simulink model "hdlcoder_led_blinking_4bit"  (R2021b)
settings: Solver=FixedStepDiscrete  StartTime=0.0  StopTime=1  RelTol=1e-3
InitFcn:
  | Ts = 1e-3;
libraries: hdlsllib x3, simulink x2
settings Model: Creator=The MathWorks, Inc.  LastModifiedBy=Jeedella
settings SolverCC: AlgebraicLoopSolver=TrustRegion
settings DataIOCC: LimitDataPoints=on  SaveFormat=Array  SaveOutput=off  SignalLogging=off  SaveTime=off  ReturnWorkspaceOutputs=off
settings OptimizationCC: BlockReduction=off  ConditionallyExecuteInputs=off  DefaultParameterBehavior=Inlined  ExpressionDepthLimit=2147483647  LifeSpan=inf
settings DebuggingCC: AlgebraicLoopMsg=error  UnderspecifiedInitializationDetection=Classic  MergeDetectMultiDrivingBlocksExec=none  SolverPrmCheckMsg=warning  SingleTaskRateTransMsg=error  ParameterPrecisionLossMsg=none  StateNameClashWarn=warning  SFUnexpectedBacktrackingDiag=warning  SFNoUnconditionalDefaultTransitionDiag=warning  SFExecutionAtInitializationDiag=none  SFMachineParentedDataDiag=warning  ArithmeticOperatorsInVariantConditions=warning
settings HardwareCC: ProdBitPerPointer=32  ProdBitPerSizeT=32  ProdBitPerPtrDiffT=32  ProdLargestAtomicFloat=None  ProdIntDivRoundTo=Undefined  ProdEndianess=Unspecified  ProdWordSize=32  ProdHWDeviceType=ASIC/FPGA->ASIC/FPGA  ProdEqTarget=off
settings ModelReferenceCC: PropagateSignalLabelsOutOfModel=off
settings SFSimCC: SimUseLocalCustomCode=off  CustomCodeUndefinedFunction=UseInterfaceOnly
settings RTWCC: RTWUseLocalCustomCode=off
settings CodeAppCC: StateflowObjectComments=on
settings GRTTargetCC: TargetLangStandard=C89/C90 (ANSI)
settings ConfigComp: CovMetricSettings=dw  CovSaveCumulativeToWorkspaceVar=on  CovSaveSingleToWorkspaceVar=on  CovExternalEMLEnable=off  CovSFcnEnable=off

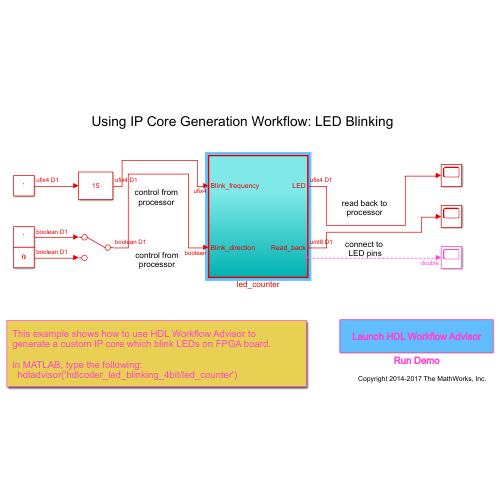
[thumbnail: Simulink's stored preview of the top-level diagram]
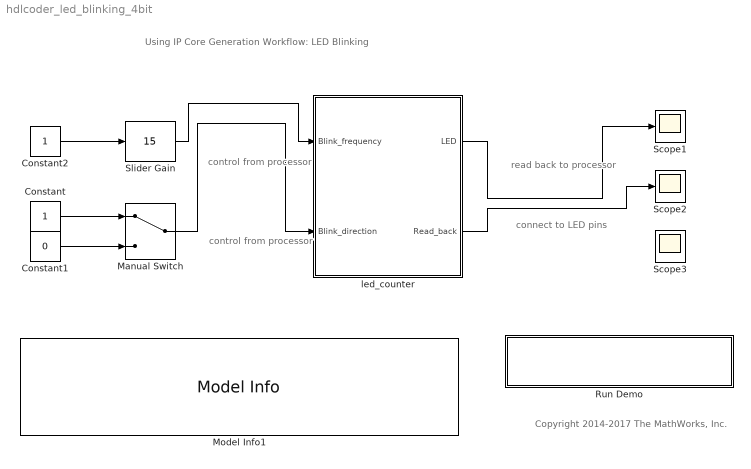
== system hdlcoder_led_blinking_4bit ==
  note: control from
      | processor
  note: Copyright 2014-2017 The MathWorks, Inc.
  note: Using IP Core Generation Workflow: LED Blinking
  note: control from
      | processor
  note: read back to
      | processor
  note: connect to
      | LED pins
  Constant : Constant  OutDataTypeStr=boolean  SampleTime=Ts
  Constant1 : Constant  Value=0  OutDataTypeStr=boolean  SampleTime=Ts
  Constant2 : Constant  OutDataTypeStr=fixdt(0, 4, 0)  SampleTime=Ts
  Manual Switch : ManualSwitch
  Model Info1 : simulink/Model-Wide Utilities/Model Info  Frame=on  DisplayStringWithTags=|  HorizontalTextAlignment=Left  LeftAlignmentValue=0.02
      | This example shows how to use HDL Workflow Advisor to    
      | generate a custom IP core which blink LEDs on FPGA board.
      |                                                          
      | In MATLAB, type the following:                           
      |   hdladvisor('hdlcoder_led_blinking_4bit/led_counter')
  Run Demo : Subsystem
      settings: OpenFcn=hdladvisor([bdroot, '/led_counter'])
      mask Display: disp('Launch HDL Workflow Advisor')
  Scope1 : Scope
  Scope2 : Scope
  Scope3 : Scope
  Slider Gain : simulink/Math Operations/Slider Gain  gain=15  low=0  high=15
  led_counter : Subsystem  TreatAsAtomicUnit=on
  wires:
  Constant/1 -> Manual Switch/1
  Constant1/1 -> Manual Switch/2
  Manual Switch/1 -> led_counter/2(Blink_direction)
  Constant2/1 -> Slider Gain/1
  Slider Gain/1 -> led_counter/1(Blink_frequency)
  led_counter/2(Read_back) -> Scope2/1
  led_counter/1(LED) -> Scope1/1
  ? -> Scope3/1

== system hdlcoder_led_blinking_4bit/Run Demo ==

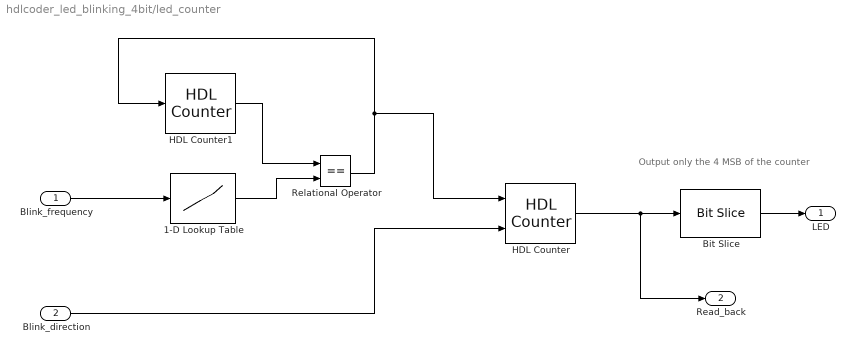
== system hdlcoder_led_blinking_4bit/led_counter ==
  note: Output only the 4 MSB of the counter
  Blink_frequency : Inport  OutDataTypeStr=fixdt(0, 4, 0)
  Blink_direction : Inport  Port=2  OutDataTypeStr=boolean
  1-D Lookup Table : Lookup_n-D  NumberOfTableDimensions=1  BreakpointsForDimension1=[0:15]  IndexSearchMethod=Evenly spaced points  Table=2.^[23:-1:8]  TableDataTypeStr=fixdt(0, 24, 0)  InterpMethod=Flat  DiagnosticForOutOfRangeInput=Error  OutDataTypeStr=fixdt(0, 24, 0)  RndMeth=Simplest  InputSameDT=on
  Bit Slice : hdlsllib/Logic and Bit Operations/Bit Slice  lidx=7  ridx=4
      settings: SourceProductBaseCode=SL
  HDL Counter : hdlsllib/Sources/HDL Counter  CountType=Free running  CountInit=0  CountStep=1  CountMax=100  CountFromType=Initial value  CountFrom=0  CountResetPort=off  CountLoadPort=off  CountEnbPort=on  CountDirPort=on  CountHitOutputPort=off  CountDataType=Unsigned  CountWordLen=8  CountFracLen=0  CountSampTime=1
  HDL Counter1 : hdlsllib/Sources/HDL Counter  CountType=Free running  CountInit=0  CountStep=1  CountMax=100  CountFromType=Initial value  CountFrom=0  CountResetPort=on  CountLoadPort=off  CountEnbPort=off  CountDirPort=off  CountHitOutputPort=off  CountDataType=Unsigned  CountWordLen=24  CountFracLen=0  CountSampTime=1
  Relational Operator : RelationalOperator  Operator===  OutDataTypeStr=boolean  RndMeth=Nearest
  LED : Outport  VectorParamsAs1DForOutWhenUnconnected=off
  Read_back : Outport  Port=2  VectorParamsAs1DForOutWhenUnconnected=off
  wires:
  HDL Counter1/1 -> Relational Operator/1
  Relational Operator/1 -> HDL Counter/1, HDL Counter1/1
  Blink_frequency/1 -> 1-D Lookup Table/1
  1-D Lookup Table/1 -> Relational Operator/2
  Blink_direction/1 -> HDL Counter/2
  Bit Slice/1 -> LED/1
  HDL Counter/1 -> Read_back/1, Bit Slice/1
